simulink model "Model"  (R2024a)
settings: Solver=VariableStepAuto  StartTime=0.0  StopTime=100  MaxStep=0.1  RelTol=1e-3
values from neighbouring files (symbols this model uses):
  c_SMA = 837.36    [params.m]
  Fmax_SMA = 10    [params.m]
  h_SMA = .3    (= 0.3)    [params.m]
  k_gn = m*g/0.01    (= 9810)    [contact3D_params.m]
  k_gt = m*g/0.1    (= 981)    [contact3D_params.m]
  m = 10    [contact3D_params.m]
  m_SMA = 0.0025    [params.m]
  max_SMA_Energy_J = 150    [params.m]
  mu_slide = 0.8    [contact3D_params.m]
  mu_stick = 0.9    [contact3D_params.m]
  n_segs = 10    [params.m]
  PWM_max = 0.35    [params.m]
  R_SMA = .08    (= 0.08)    [params.m]
  r_SMA2limb = 0.009    [params.m]
  swing_angle = swing_angles(i)    [params.m]
  T_amb = 23    [params.m]
  V_0 = 7    [params.m]
  v_gn_max = 0.03    [contact3D_params.m]
  v_gt_max = 0.03    [contact3D_params.m]
  vLimit = 0.01    [contact3D_params.m]
undefined symbols (not defined in the file or in its folder): Newton, Raphson, X, Y, Z
libraries: sm_lib x223, nesl_utility x184, simulink x24, simulink_extras x6
(part 16 of 16)

== matlab function Model/MATLAB Function ==
  data: p0 input; xfl output; yfl output; xcl output; ycl output; xbl output; ybl output; xfr output; yfr output; xcr output; ycr output; xbr output; ybr output; p1 input; p2 input; p3 input; p4 input; p5 input; p6 input; p7 input; swing_angle input
function [xfl, yfl, xcl, ycl, xbl, ybl, xfr, yfr, xcr, ycr, xbr, ybr]= walk(p0, p1, p2, p3, p4, p5, p6, p7, swing_angle)


in = 20;
out = 30;
forward = swing_angle;
backward = -swing_angle;

if (p0 == 1) % start
    xfl = 0;
    xbl = 0;
    xcr = 0;
    xcl = 0;
    xfr = 0;
    xbr = 0;
    yfl = 0;
    ybl = 0;
    ycr = 0;
    ycl = 0;
    yfr = 0;
    ybr = 0;

elseif (p1 == 1) % legs out
    xfl = 0;
    xbl = 0;
    xcr = 0;
    xcl = 0;
    xfr = 0;
    xbr = 0;
    yfl = -in;
    ybl = -in;
    ycr = in;
    ycl = out;
    yfr = -out;
    ybr = -out;


elseif (p2 == 1) % legs out and forward/back
    xfl = backward;
    xbl = backward;
    xcr = backward;
    xcl = forward;
    xfr = forward;
    xbr = forward;
    yfl = -in;
    ybl = -in;
    ycr = in;
    ycl = out;
    yfr = -out;
    ybr = -out;

elseif (p3 == 1) % stand again
    xfl = backward;
    xbl = backward;
    xcr = backward;
    xcl = forward;
    xfr = forward;
    xbr = forward;
    yfl = -in;
    ybl = -in;
    ycr = in;
    ycl = -in;
    yfr = in;
    ybr = in;

elseif (p4 == 1) % lift other legs
    xfl = backward;
    xbl = backward;
    xcr = backward;
    xcl = forward;
    xfr = forward;
    xbr = forward;
    yfl = out;
    ybl = out;
    ycr = -out;
    ycl = -in;
    yfr = in;
    ybr = in;

elseif (p5 == 1) % move forward
    xfl = forward;
    xbl = forward;
    xcr = forward;
    xcl = backward;
    xfr = backward;
    xbr = backward;
    yfl = out;
    ybl = out;
    ycr = -out;
    ycl = -in;
    yfr = in;
    ybr = in;

elseif (p6 == 1) % stand again
    xfl = forward;
    xbl = forward;
    xcr = forward;
    xcl = backward;
    xfr = -backward;
    xbr = -backward;
    yfl = -in;
    ybl = -in;
    ycr = in;
    ycl = -in;
    yfr = in;
    ybr = in;   

elseif(p7 ==1) % replaces p1 in loop
    xfl = forward;
    xbl = forward;
    xcr = forward;
    xcl = backward;
    xfr = -backward;
    xbr = -backward;
    yfl = -in;
    ybl = -in;
    ycr = in;
    ycl = out;
    yfr = -out;
    ybr = -out;
else
    xfl = 0;
    xbl = 0;
    xcr = 0;
    xcl = 0;
    xfr = 0;
    xbr = 0;
    yfl = 0;
    ybl = 0;
    ycr = 0;
    ycl = 0;
    yfr = 0;
    ybr = 0;
end



% xfl = 0;
% xbl = 0;
% xcr = 0;
% xcl = 0;
% xfr = 0;
% xbr = 0;
% yfl = -10;
% ybl = -10;
% ycr = 0;
% ycl = 30;
% yfr = -30;
% ybr = -30;

== matlab function Model/LIMB 1: Center LEFT/Limb 1/SMA4 F(V)/F(T) ==
  data: T input; F output; Fmax_SMA input
function F = fcn(T, Fmax_SMA)

% INPUT: Temperature (C), max SMA force
% OUTPUT: Force [N]

% Based around T_transition = 90C

% THOS WHOLE RELATIONSHIP NEEDS IMPROVEMENT, LOOSELY BASED ON fig 6b from:
% https://link.springer.com/article/10.1007/s11340-024-01059-9 and 
% https://www.dynalloy.com/pdfs/TCF1140_2.pdf
if T>110
    F = Fmax_SMA;
elseif T>95
    F = Fmax_SMA - 0.2*Fmax_SMA * ((110-T)/15);
elseif T>85
    F = 0.8*Fmax_SMA - 0.55*Fmax_SMA * ((95-T)/10);
else
    F = 0.25*Fmax_SMA - 0.25*Fmax_SMA * ((85-T)/50);
end

== matlab function Model/LIMB 1: Center LEFT/BANG-BANG CONTROLLER ==
  data: theta_X input; D1 output; theta_Y input; D2 output; D3 output; D4 output; Target_X input; Target_Y input; PWM_max input
function [D1, D2, D3, D4] = fcn(theta_X, theta_Y, Target_X, Target_Y, PWM_max)

    % INPUT: Rotations about -X and -Y axes, Target angles, max PWM
    % OUTPUT: Duty Cycles:
    %   D1: +X rotation
    %   D2: -X rotation
    %   D3: +Y rotation
    %   D4: -Y rotation

    X_err = Target_X - theta_X;
    Y_err = Target_Y - theta_Y;

    D1 = 0; D2 = 0; D3 = 0; D4 = 0;

    if X_err > 5
        D1 = PWM_max;
    elseif X_err > 1
        D1 = PWM_max / 1.5;
    elseif X_err < -5
        D2 = PWM_max;
    elseif X_err < -1
        D2 = PWM_max / 1.5;
    end

    if Y_err > 5
        D3 = PWM_max;
    elseif Y_err > 1
        D3 = PWM_max / 1.5;
    elseif Y_err < -5
        D4 = PWM_max;
    elseif Y_err < -1
        D4 = PWM_max / 1.5;
    end

== matlab function Model/LIMB 1: Center LEFT/Limb 1/MATLAB Function1 ==
  data: R input; alpha_xz output; alpha_yz output; alpha_xy output
function [alpha_xz, alpha_yz, alpha_xy] = orientation_to_plane_angles(R)
% ORIENTATION_TO_PLANE_ANGLES Convert orientation to angle projections on XZ, YZ, XY planes
%   Inputs:
%       R - Rotation Matrix
%   Outputs:
%       alpha_xz - Angle in radians on the XZ-plane
%       alpha_yz - Angle in radians on the YZ-plane
%       alpha_xy - Angle in radians on the XY-plane
    
    % Define the local forward vector (local Z-axis)
    v_local = [0; 0; 1];
    
    % Transform to global coordinates
    v_global = R * v_local;
    
    % Projection onto XZ-plane
    v_xz = [v_global(1); 0; v_global(3)];
    alpha_xz = rad2deg(-(atan2(v_xz(3), v_xz(1)) - pi/2));
    
    % Projection onto YZ-plane
    v_yz = [0; v_global(2); v_global(3)];
    alpha_yz = rad2deg(atan2(v_yz(3), v_yz(2)) - pi/2);
    
    % Projection onto XY-plane
    v_xy = [v_global(1); v_global(2); 0];
    alpha_xy = rad2deg(atan2(v_xy(2), v_xy(1)) + pi/4);
end

== matlab function Model/LIMB 1: Center LEFT/PID CONTROLLER ==
  data: eX input; deX input; seX input; D1 output; eY input; D2 output; D3 output; D4 output; deY input; seY input; PWM_max input
function [D1, D2, D3, D4] = fcn(eX, deX, seX, eY, deY, seY, PWM_max)

    % INPUT: errors and derivatives about -x and -y axes, max PWM
    % OUTPUT: Duty Cycles:

    kp = 0.5;
    kd = 0;
    ki = 0.05;

    D1 = 0; D2 = 0; D3 = 0; D4 = 0;

    if eX > 0.5
        D1 = min((kp*eX + kd*deX + ki*seX), PWM_max);
    elseif eX < -0.5
        D2 = min((kp*-eX + kd*-deX + ki*-seX), PWM_max);
    end

    if eY > 0.5
        D3 = min((kp*eY + kd*deY + ki*seY), PWM_max);
    elseif eY < -0.5
        D4 = min((kp*-eY + kd*-deY + ki*-seY), PWM_max);
    end

== matlab function Model/LIMB 1: Back RIGHT/BANG-BANG CONTROLLER ==
  data: theta_X input; D1 output; theta_Y input; D2 output; D3 output; D4 output; Target_X input; Target_Y input; PWM_max input
function [D1, D2, D3, D4] = fcn(theta_X, theta_Y, Target_X, Target_Y, PWM_max)

    % INPUT: Rotations about -X and -Y axes, Target angles, max PWM
    % OUTPUT: Duty Cycles:
    %   D1: +X rotation
    %   D2: -X rotation
    %   D3: +Y rotation
    %   D4: -Y rotation

    X_err = Target_X - theta_X;
    Y_err = Target_Y - theta_Y;

    D1 = 0; D2 = 0; D3 = 0; D4 = 0;

    if X_err > 5
        D1 = PWM_max;
    elseif X_err > 1
        D1 = PWM_max / 1.5;
    elseif X_err < -5
        D2 = PWM_max;
    elseif X_err < -1
        D2 = PWM_max / 1.5;
    end

    if Y_err > 5
        D3 = PWM_max;
    elseif Y_err > 1
        D3 = PWM_max / 1.5;
    elseif Y_err < -5
        D4 = PWM_max;
    elseif Y_err < -1
        D4 = PWM_max / 1.5;
    end
